simulink model "DifferentialDriveSMCModel"  (R2020b)
settings: Solver=VariableStepAuto  StartTime=0.0  StopTime=120  RelTol=1e-3
undefined symbols (not defined in the file): beta, k, ki, l, L, r, vx
libraries: simulink_extras x2, simulink x1
settings Model: Creator=김예온  LastModifiedBy=USER
settings SolverCC: ZeroCrossAlgorithm=Adaptive
settings DebuggingCC: IgnoredZcDiagnostic=none

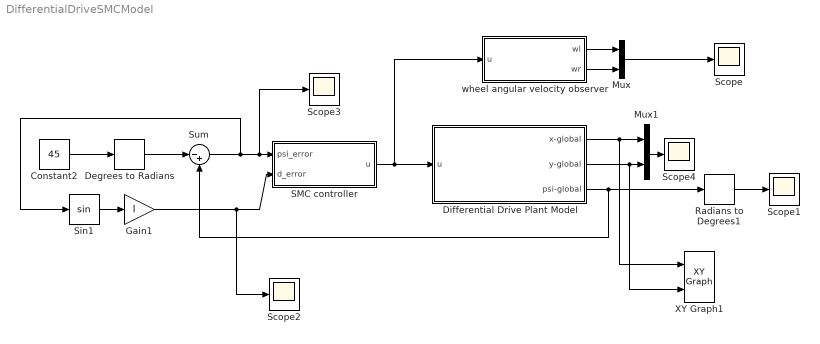
== system DifferentialDriveSMCModel ==
  Constant2 : Constant  Value=45
  Degrees to Radians : simulink_extras/Transformations/Degrees to Radians
  Differential Drive Plant Model : Subsystem
  Gain1 : Gain  Gain=l
  Mux : Mux  Inputs=2
  Mux1 : Mux  Inputs=2
  Radians to Degrees1 : simulink_extras/Transformations/Radians to Degrees
  SMC controller : Subsystem
  Scope{,1..4} (5 alike) : Scope
  Sin1 : Trigonometry
  Sum : Sum  Inputs=|-+
  XY Graph1 : simulink/Sinks/XY Graph  xmin=-1  xmax=10  ymin=-10  ymax=10  st=-1
  wheel angular velocity observer : Subsystem
  wires:
  SMC controller/1(u) -> wheel angular velocity observer/1(u), Differential Drive Plant Model/1(u)
  wheel angular velocity observer/1(wl) -> Mux/1
  wheel angular velocity observer/2(wr) -> Mux/2
  Differential Drive Plant Model/1(x-global) -> XY Graph1/1, Mux1/1
  Differential Drive Plant Model/2(y-global) -> XY Graph1/2, Mux1/2
  Mux/1 -> Scope/1
  Radians to Degrees1/1 -> Scope1/1
  Differential Drive Plant Model/3(psi-global) -> Radians to Degrees1/1, Sum/2
  Constant2/1 -> Degrees to Radians/1
  Degrees to Radians/1 -> Sum/1
  Sin1/1 -> Gain1/1
  Sum/1 -> Sin1/1, Scope3/1, SMC controller/1(psi_error)
  Gain1/1 -> Scope2/1, SMC controller/2(d_error)
  Mux1/1 -> Scope4/1

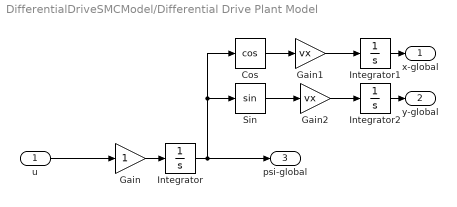
== system DifferentialDriveSMCModel/Differential Drive Plant Model ==
  u : Inport
  Cos : Trigonometry  Operator=cos
  Gain : Gain
  Gain1 : Gain  Gain=vx
  Gain2 : Gain  Gain=vx
  Integrator : Integrator
  Integrator1 : Integrator
  Integrator2 : Integrator
  Sin : Trigonometry
  x-global : Outport
  y-global : Outport  Port=2
  psi-global : Outport  Port=3
  wires:
  Gain/1 -> Integrator/1
  u/1 -> Gain/1
  Integrator/1 -> Cos/1, Sin/1, psi-global/1
  Integrator1/1 -> x-global/1
  Integrator2/1 -> y-global/1
  Gain1/1 -> Integrator1/1
  Cos/1 -> Gain1/1
  Sin/1 -> Gain2/1
  Gain2/1 -> Integrator2/1

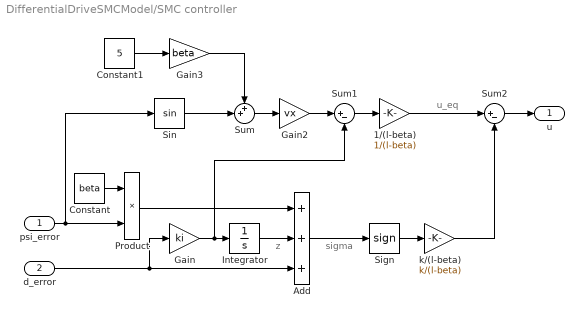
== system DifferentialDriveSMCModel/SMC controller ==
  note: sigma
  note: u_eq
  note: z
  psi_error : Inport
  d_error : Inport  Port=2
  1/(l-beta) : Gain  Gain=1/(l-beta)
  Add : Sum  Inputs=+++
  Constant : Constant  Value=beta
  Constant1 : Constant  Value=5
  Gain : Gain  Gain=ki
  Gain2 : Gain  Gain=vx
  Gain3 : Gain  Gain=beta
  Integrator : Integrator
  Product : Product
  Sign : Signum  ZeroCross=off
  Sin : Trigonometry
  Sum : Sum  Inputs=++|
  Sum1 : Sum  Inputs=|+-
  Sum2 : Sum  Inputs=|+-
  k/(l-beta) : Gain  Gain=k/(l-beta)
  u : Outport
  wires:
  Constant/1 -> Product/1
  psi_error/1 -> Sin/1, Product/2
  d_error/1 -> Add/3, Gain/1
  Gain/1 -> Sum1/2, Integrator/1
  Product/1 -> Add/1
  Integrator/1 -> Add/2
  Sin/1 -> Sum/2
  Gain3/1 -> Sum/1
  Sum/1 -> Gain2/1
  Gain2/1 -> Sum1/1
  Sum1/1 -> 1/(l-beta)/1
  Add/1 -> Sign/1
  Sign/1 -> k/(l-beta)/1
  1/(l-beta)/1 -> Sum2/1
  Sum2/1 -> u/1
  k/(l-beta)/1 -> Sum2/2
  Constant1/1 -> Gain3/1

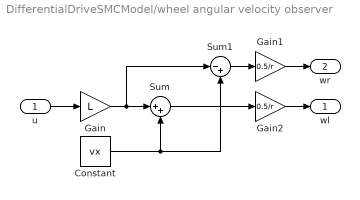
== system DifferentialDriveSMCModel/wheel angular velocity observer ==
  u : Inport
  Constant : Constant  Value=vx
  Gain : Gain  Gain=L
  Gain1 : Gain  Gain=0.5/r
  Gain2 : Gain  Gain=0.5/r
  Sum : Sum  Inputs=|++
  Sum1 : Sum  Inputs=|-+
  wl : Outport
  wr : Outport  Port=2
  wires:
  u/1 -> Gain/1
  Gain/1 -> Sum1/1, Sum/1
  Constant/1 -> Sum1/2, Sum/2
  Sum1/1 -> Gain1/1
  Gain2/1 -> wl/1
  Sum/1 -> Gain2/1
  Gain1/1 -> wr/1
